simulink subsystem "pololu_37D_torque_first_order"  (R2023b)
settings: Solver=VariableStepAuto  StartTime=0.0  StopTime=10.0  RelTol=1e-3
model mask{L=2.3e-3, R=2.1, K=1.32}
  mask prompts: L "Inductance"; R "Resistance"; K "Motor Constant"
settings Model: Creator=kiraa  LastModifiedBy=kiraa

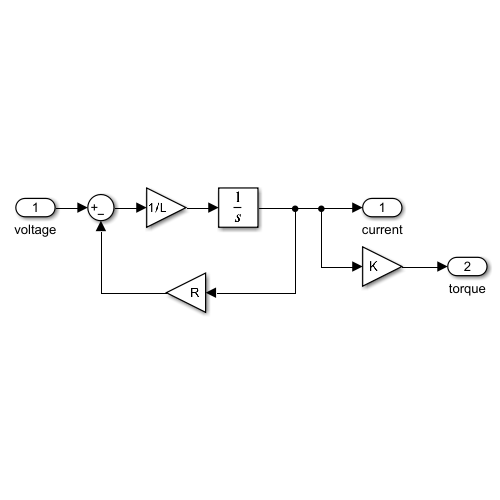
[thumbnail: Simulink's stored preview of the top-level diagram]
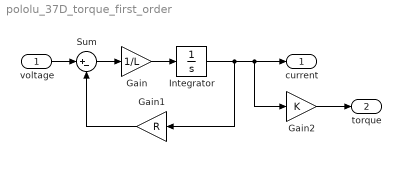
== system pololu_37D_torque_first_order ==
  voltage : Inport
  Gain : Gain  Gain=1/L
  Gain1 : Gain  Gain=R
  Gain2 : Gain  Gain=K
  Integrator : Integrator
  Sum : Sum  Inputs=|+-
  current : Outport
  torque : Outport  Port=2
  wires:
  Gain/1 -> Integrator/1
  Integrator/1 -> Gain2/1, current/1, Gain1/1
  Gain1/1 -> Sum/2
  Sum/1 -> Gain/1
  voltage/1 -> Sum/1
  Gain2/1 -> torque/1
